simulink model "assignment_block_1_2019v"  (R2019b)
settings: Solver=VariableStepAuto  StartTime=0.0  StopTime=10.0  RelTol=1e-3
undefined symbols (not defined in the file or in its folder): sigbuilder_block
settings Model: Creator=Brigosha_Guest  LastModifiedBy=Brigosha_Guest
settings DebuggingCC: UnconnectedInputMsg=none  UnconnectedOutputMsg=none  UnconnectedLineMsg=none  SFMachineParentedDataDiag=error
settings ModelReferenceCC: EnableRefExpFcnMdlSchedulingChecks=off
settings RTWCC: Description=Generic Real-Time Target

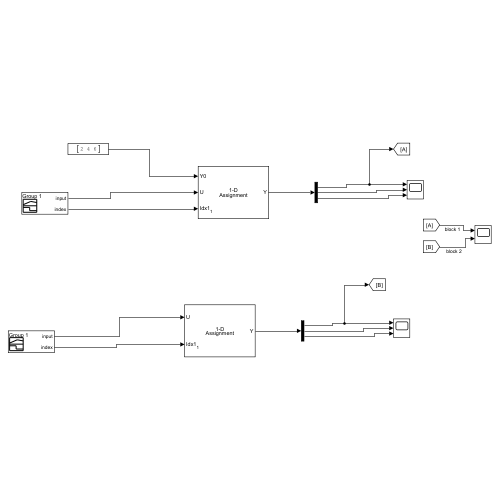
[thumbnail: Simulink's stored preview of the top-level diagram]
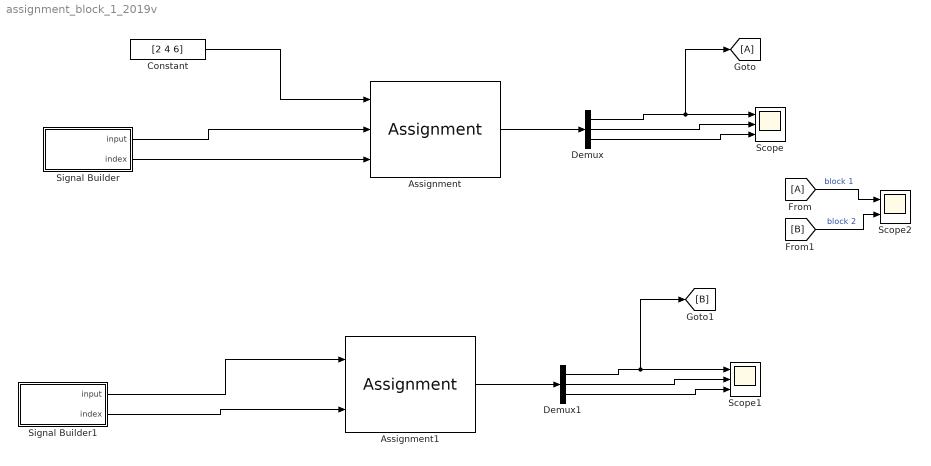
== system assignment_block_1_2019v ==
  Assignment : Assignment  DiagnosticForDimensions=Warning  IndexOptions=Index vector (port)  Indices=1  OutputSizes=1
  Assignment1 : Assignment  OutputInitialize=Specify size for each dimension in table  DiagnosticForDimensions=Warning  IndexOptions=Index vector (port)  Indices=1  OutputSizes=3
  Constant : Constant  Value=[2 4 6]
  Demux : Demux  Outputs=3
  Demux1 : Demux  Outputs=3
  Scope : Scope  NumInputPorts=3
  Scope1 : Scope  NumInputPorts=3
  Scope2 : Scope  NumInputPorts=2
  Signal Builder : Subsystem  Tag=STV Subsys  LoadFcn=sigbuilder_block('load');  StartFcn=sigbuilder_block('start');  StopFcn=sigbuilder_block('stop');  ClipboardFcn=sigbuilder_block('clipboard');  mask(Sigbuilder block){tuvar=[0:10]}
      mask help: Simulink:masks:SigbuilderBlock_MD
      mask init:
      | if ~strcmp(get_param(bdroot(gcbh),'SimulationStatus'),'stopped') tuvar = sigbuilder_block('maskInit'); end
      settings: CopyFcn=sigbuilder_block('copy');  DeleteFcn=sigbuilder_block('delete');  ModelCloseFcn=sigbuilder_block('modelClose');  PreSaveFcn=sigbuilder_block('preSave');  PauseFcn=sigbuilder_block('pause');  ContinueFcn=sigbuilder_block('continue');  NameChangeFcn=sigbuilder_block('namechange');  OpenFcn=sigbuilder_block('open',[437.6 153 550.4 359.25 ]);  CloseFcn=sigbuilder_block('close');
      mask Display: plot(0, 0, 100, 100,[2, 2, 32, 32, 2], [68, 8, 8, 68, 68],[32, 2], [38, 38], [32, 19, 2],[53, 60, 44], [32, 17, 17, 2],[16, 16, 31, 31]);txt = getActiveGroup(gcbh);text(2, 100, txt,'verticalAlignment', 'top');
  Signal Builder1 : Subsystem  Tag=STV Subsys  LoadFcn=sigbuilder_block('load');  StartFcn=sigbuilder_block('start');  StopFcn=sigbuilder_block('stop');  ClipboardFcn=sigbuilder_block('clipboard');  mask(Sigbuilder block){tuvar=[0:10]}
      mask help: Simulink:masks:SigbuilderBlock_MD
      mask init:
      | if ~strcmp(get_param(bdroot(gcbh),'SimulationStatus'),'stopped') tuvar = sigbuilder_block('maskInit'); end
      settings: CopyFcn=sigbuilder_block('copy');  DeleteFcn=sigbuilder_block('delete');  ModelCloseFcn=sigbuilder_block('modelClose');  PreSaveFcn=sigbuilder_block('preSave');  PauseFcn=sigbuilder_block('pause');  ContinueFcn=sigbuilder_block('continue');  NameChangeFcn=sigbuilder_block('namechange');  OpenFcn=sigbuilder_block('open',[437.6 153 550.4 359.25 ]);  CloseFcn=sigbuilder_block('close');
      mask Display: plot(0, 0, 100, 100,[2, 2, 32, 32, 2], [68, 8, 8, 68, 68],[32, 2], [38, 38], [32, 19, 2],[53, 60, 44], [32, 17, 17, 2],[16, 16, 31, 31]);txt = getActiveGroup(gcbh);text(2, 100, txt,'verticalAlignment', 'top');
  wires:
  Constant/1 -> Assignment/1
  Assignment/1 -> Demux/1
  Signal Builder/1(input) -> Assignment/2
  Signal Builder/2(index) -> Assignment/3
  Demux/1 -> [A], Scope/1
  Demux/2 -> Scope/2
  Demux/3 -> Scope/3
  Demux1/3 -> Scope1/3
  Demux1/2 -> Scope1/2
  Signal Builder1/2(index) -> Assignment1/2
  Signal Builder1/1(input) -> Assignment1/1
  Assignment1/1 -> Demux1/1
  Demux1/1 -> [B], Scope1/1
  [A] -> Scope2/1  "block 1"
  [B] -> Scope2/2  "block 2"

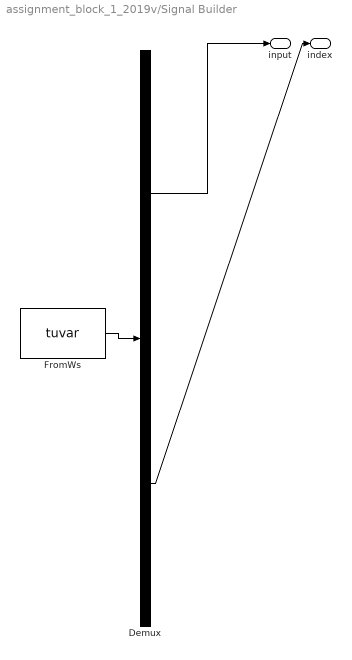
== system assignment_block_1_2019v/Signal Builder ==
  Demux : Demux  Tag=STV Demux  Outputs=2
      settings: DisplayOption=none
  FromWs : FromWorkspace  Tag=STV FromWs  VariableName=tuvar
      SigBuilderData=|
      | common.afterFinalStr = 'Extrapolate'
      | common.sampleTime = 0
      | dataSet.timeRange = [0 10]
      | dataSet.name = 'Group 1'
      | sbobj.Groups.Name = 'Group 1'
      | sbobj.Groups.Signals(1).Name = 'input'
      | sbobj.Groups.Signals(1).XData = [0 1 2 3 4 5 6 7 8 9 10]
      | sbobj.Groups.Signals(1).YData = [0 10 20 30 40 50 60 70 80 90 100]
      | sbobj.Groups.Signals(2).Name = 'index'
      | sbobj.Groups.Signals(2).XData = [0 1 1 2 2 3 3 4 4 5 5 6 7 7 8 8 9 9 10]
      | sbobj.Groups.Signals(2).YData = [3 3 1 1 2 2 1 1 3 3 2 2 2 3 3 1 1 3 3]
  input : Outport  Tag=STV Outport
  index : Outport  Tag=STV Outport  Port=2
  wires:
  Demux/1 -> input/1
  FromWs/1 -> Demux/1
  Demux/2 -> index/1

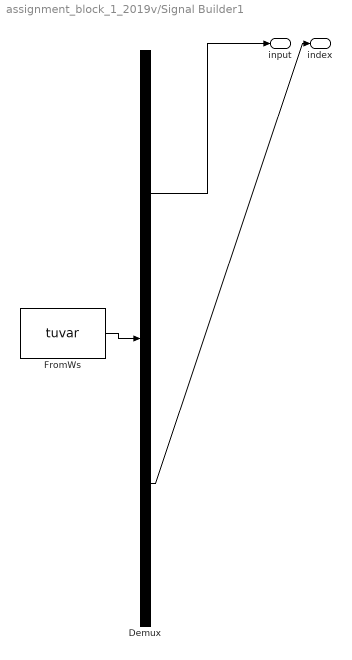
== system assignment_block_1_2019v/Signal Builder1 ==
  Demux : Demux  Tag=STV Demux  Outputs=2
      settings: DisplayOption=none
  FromWs : FromWorkspace  Tag=STV FromWs  VariableName=tuvar
      SigBuilderData=|
      | common.afterFinalStr = 'Extrapolate'
      | common.sampleTime = 0
      | dataSet.timeRange = [0 10]
      | dataSet.name = 'Group 1'
      | sbobj.Groups.Name = 'Group 1'
      | sbobj.Groups.Signals(1).Name = 'input'
      | sbobj.Groups.Signals(1).XData = [0 1 2 3 4 5 6 7 8 9 10]
      | sbobj.Groups.Signals(1).YData = [0 10 20 30 40 50 60 70 80 90 100]
      | sbobj.Groups.Signals(2).Name = 'index'
      | sbobj.Groups.Signals(2).XData = [0 1 1 2 2 3 3 4 4 5 5 6 7 7 8 8 9 9 10]
      | sbobj.Groups.Signals(2).YData = [3 3 1 1 2 2 1 1 3 3 2 2 2 3 3 1 1 3 3]
  input : Outport  Tag=STV Outport
  index : Outport  Tag=STV Outport  Port=2
  wires:
  Demux/2 -> index/1
  FromWs/1 -> Demux/1
  Demux/1 -> input/1
